simulink model "control1_flatness"  (R2023b)
settings: Solver=VariableStepAuto  StartTime=0.0  StopTime=8  RelTol=1e-3
values from neighbouring files (symbols this model uses):
  d = obs_r+threshold    (= 0.3)    [main.m]
  damping_coeff = 1/sqrt(2)    [main.m]
  initial_position = [0,r]    [main.m]
  natural_frequency = 10    [main.m]
  obs_r = 0.1    [main.m]
  obs_x = [20]    [main.m]
  obs_y = [20]    [main.m]
  parking_position = [0,0]    [main.m]
  r = 1    [main.m]
  T = 2*pi    (= 6.28318530718)    [main.m]
  t_values = 0:dt:T*1.1    [main.m]
  threshold = 0.2    [main.m]
(part 3 of 3)

== matlab function control1_flatness/Trajectory generator/Trajectory generator and obstacle detection1/Subsystem1/Whole trajectory calculation + flatness ==
  data: r input; trajectory_x output; t_values input; T input; trajectory_y output; v_d_array output; omega_d_array output; theta_d_array output; recalculate output; recalculate_obs input; d input; blending input; theta11 input; xd input; yd input; recalculate_obs1 output; old_trajectory_x input; old_trajectory_y input
function [trajectory_x, trajectory_y, v_d_array, omega_d_array, theta_d_array, recalculate,recalculate_obs1]  = fcn( r, t_values,T, recalculate_obs,d, blending, theta11, xd, yd,old_trajectory_x, old_trajectory_y)
    x0 = 0;
    y0 = 1;
    W = 2;
    H = 2;
    R = H / 2; 
    xc = x0 + W; 
    yc = y0 + R;      
    if(~recalculate_obs)
        trajectory_x = zeros(length(t_values), 1);
        trajectory_y = ones(length(t_values), 1);
        % Parameters

        
        for i = 1:length(t_values)
            t = t_values(i);
            
            if t < T/4
                % Move right
                trajectory_x(i) = x0 + (W/T*4) * t;
                trajectory_y(i) = y0;
                
            elseif t < T/2
                % Move up
                theta = -pi/2 + pi * (t - T/4) / (T/4);  % Angle from -pi/2 to pi/2
                trajectory_x(i) = xc + R * cos(theta);  % Half-circle x
                trajectory_y(i) = yc + R * sin(theta);  % Half-circle y
                
            elseif t < 3*T/4
                % Move left
                trajectory_x(i) = x0 + W - (W/T*4) * (t - T/2);
                trajectory_y(i) = y0 + H;
                
            elseif t< T
                % Move down
                trajectory_x(i) = x0;
                trajectory_y(i) = y0 + H - (H/T*4) * (t - 3*T/4);
            else
                trajectory_x(i) = x0;
                trajectory_y(i) = y0;
            end
        end

    else
        % Obstacle was detected: in the point x, y with angle theta
        center_trajectory = [x0+W/2, y0+H/2];
        % Loading previous version of the trajectory 
        % to avoid additional and useless computations of
        % previous desired path
        trajectory_x = old_trajectory_x;
        trajectory_y = old_trajectory_y;
        x1 = xd;
        y1 = yd;
        points = [trajectory_x,trajectory_y];
        [~, start_idx] = min(vecnorm(points - [x1,y1], 2, 2));

        theta1 = -theta11+pi/2;  % Adjusting the angle to get the anglefrom vertical axis (theta11 is wrt horisontal axis)

        % Estimate the obstacle location
        theta_range = linspace(theta1 - pi/4, theta1 + pi/4, 300);
        x_arc = x1 + d * sin(theta_range);
        y_arc = y1 + d * cos(theta_range);



        % Loop through the trajectory points to check for intersections

        obs_x = x1;
        obs_y = y1;
        obs_idx = start_idx;
        for i = start_idx:length(trajectory_x) - 1
            x_traj_seg = [trajectory_x(i), trajectory_x(i + 1)];
            y_traj_seg = [trajectory_y(i), trajectory_y(i + 1)];
            
            for j = 1:length(x_arc) - 1
                x_arc_seg = [x_arc(j), x_arc(j + 1)];
                y_arc_seg = [y_arc(j), y_arc(j + 1)];
                
                % Check if the two segments intersect
                [intersects, ix, iy] = segmentIntersection(x_traj_seg, y_traj_seg, x_arc_seg, y_arc_seg);
        
                if intersects
                    % Intersection found, assign coordinates
                    obs_x = ix;
                    obs_y = iy;
                    obs_idx = i;
                    break; % Exit the loop once intersection is found
                end
             end
            if obs_x ~= x1
                break; 
            end
        end
        % -- > Finding the point where the obstacle avoidance trajectory should 
        % be finished, point from which the robot should continue on
        % the regular trajectory.Creating a circle of radius d, with the 
        % center in [center_obs_x, center_obs_y].
        % After that, finding an intersection of that circle with the 
        % previous trajectory.
    
        theta_values = linspace(0, 2*pi, 500);
        x_circle = obs_x + d * cos(theta_values);
        y_circle = obs_y + d * sin(theta_values);

        % Loop through the trajectory points to check for intersections

        x2 = x1;
        y2 = y1;
        end_idx_trajectory = obs_idx;
        end_idx_circle = 1;

        for i = obs_idx:length(trajectory_x) - 1
            x_traj_seg = [trajectory_x(i), trajectory_x(i + 1)];
            y_traj_seg = [trajectory_y(i), trajectory_y(i + 1)];
            
            for j = 1:length(x_circle) - 1
                x_circle_seg = [x_circle(j), x_circle(j + 1)];
                y_circle_seg = [y_circle(j), y_circle(j + 1)];
                
                % Check if the two segments intersect
                [intersects, ix, iy] = segmentIntersection(x_traj_seg, y_traj_seg, x_circle_seg, y_circle_seg);
        
                if intersects
                    % Intersection found, assign coordinates
                    x2 = ix;
                    y2 = iy;
                    end_idx_trajectory = i;
                    end_idx_circle = j;
                    break; 
                end
            end
            if x2 ~= x1, break; end
        end

        % --> Finding the longer arc of the circle around obstacle
        % This will be the desired obstacle avoidance path
        points = [x_circle' y_circle']; % Nx2 array
        [~, idx1] = min(vecnorm(points - [x1,y1], 2, 2));
        idx2 = end_idx_circle;
        
        if idx1 < idx2
            arc1 = points(idx1:idx2, :);       
            arc2 = [points(idx2:end, :); points(1:idx1, :)];
        else
            arc1 = points(idx2:idx1, :);       
            arc2 = [points(idx1:end, :); points(1:idx2, :)];
        end
        
        idx_point1 = floor(size(arc1,1)/2);
        idx_point2 = floor(size(arc2,1)/2);
        
        distance1 = (arc1(idx_point1,1)-center_trajectory(1))^2+(arc1(idx_point1,2)-center_trajectory(2))^2;
        distance2 =  (arc2(idx_point2,1)-center_trajectory(1))^2+(arc2(idx_point2,2)-center_trajectory(2))^2;
        
        if distance1>distance2
            longer_arc = arc1;
        else
            longer_arc = arc2;
        end
        % Reverse if needed
        if(abs(longer_arc(1,1)-x1)>abs(longer_arc(1,1)-x2))
            longer_arc = flip(longer_arc);
        end


        % --> Creating a new trajectory
        idx1 = start_idx;
        idx2 = end_idx_trajectory;
        % Change of the trajectory is allowed if the ordering is okay
        % first indexwise is the point of detection and then the obstacle
        % (should always be satisfied)
        if(idx1<idx2 && t_values(idx2)<T)

            n_points = idx2 - idx1 + 1;
            total_points = size(longer_arc,1);
            indices = round(linspace(1, total_points, n_points));
            % Smoothly blend the two trajectories if needed
            trajectory_avoid_x = longer_arc(indices,1);
            trajectory_avoid_y = longer_arc(indices,2);
            trajectory_old_x = trajectory_x(idx1:idx2);
            trajectory_old_y = trajectory_y(idx1:idx2);

            trajectory_x(idx1:idx2) = blending*trajectory_avoid_x + (1-blending)*trajectory_old_x;
            trajectory_y(idx1:idx2) = blending*trajectory_avoid_y + (1-blending)*trajectory_old_y;

        end
    end

    recalculate_obs1 = 0;
    recalculate = 0;


    dt = t_values(2) - t_values(1);

    %  Derivatives
    dx_d = gradient(trajectory_x, dt);
    dy_d = gradient(trajectory_y, dt);
    ddx_d = gradient(dx_d, dt);
    ddy_d = gradient(dy_d, dt);
    
    v_d_array = sqrt(dx_d.^2 + dy_d.^2);
    omega_d_array = (ddy_d .* dx_d - ddx_d .* dy_d) ./ ((dx_d.^2 + dy_d.^2)+eps);
    theta_d_array=atan2(dy_d,dx_d);

end

== matlab function control1_flatness/One circle detection/one circle detection ==
  data: t input; x input; regulation_flag output; y input; initial_position input; regulation_flag_previous input; constant input
function regulation_flag = fcn( t, x,y,initial_position, regulation_flag_previous, constant)
if(regulation_flag_previous==0)
    if (abs(initial_position(1)- x)<0.001 && abs(initial_position(2)-y)<0.001 &&(t>constant))
        regulation_flag=1;
    else 
        regulation_flag=0;
    end
else
    regulation_flag =1;
end

== matlab function control1_flatness/Trajectory generator/Trajectory generator and obstacle detection1/Subsystem3/Triggered Subsystem/MATLAB Function1 ==
  data: t input; t_values input; trajectory_x input; x_d output; trajectory_y input; y_d output; v_d output; omega_d output; theta_d output; v_d_array input; omega_d_array input; theta_d_array input; i input; new_i output
function [x_d, y_d, v_d, omega_d, theta_d, new_i] = fcn(t, t_values, trajectory_x, trajectory_y, v_d_array, omega_d_array, theta_d_array,i)

    % When the block is not enabled (on the start),this is used to give initial position
    if (i==0)
        new_i=1;
    else
        new_i =i;
    end

    [~, idx] = min(abs(t_values - t));  % closest index to current time
    if(t>t_values(end))
        idx = length(t_values);
    end
    % Position
    x_d = trajectory_x(idx);  
    y_d = trajectory_y(idx);

    % Flatness
    v_d = v_d_array(idx);  
    omega_d = omega_d_array(idx);
    theta_d = theta_d_array(idx);

== matlab function control1_flatness/General control scheme with flatness1/Calculation of e1, e2, and e3 ==
  data: e_x input; e1 output; e_y input; e_theta input; e2 output; e3 output; theta input
function [e1,e2,e3] = fcn(e_x,e_y,e_theta,theta)
e1=e_x*cos(theta)+e_y*sin(theta);
e2=-e_x*sin(theta)+e_y*cos(theta);

if (abs(e_theta)>=2*pi)
   e_theta = mod(e_theta -2*pi, 2*pi);
end
if (abs(e_theta)>=pi)
   e_theta = mod(e_theta + pi, 2*pi)-pi;
end

e3=e_theta;
end

== matlab function control1_flatness/General control scheme with flatness1/MATLAB Function ==
  data: a input; u1 output; dam_cof input; e1 input; e2 input; e3 input; v_d input; omega_d input; u2 output
function [u1,u2] = controller(a,dam_cof,e1,e2,e3,v_d,omega_d)
k1=2*dam_cof*a
k3=k1
if abs(v_d)<1e-4
    if v_d>=0
        v_d=1e-4;
    else
        v_d=-1e-4;
    end
end
k2=(a^2-(omega_d^2))/v_d % v_d is constant for circular motion,while omega_d constant(diffrent from zero)
u1=-k1*e1;
u2=-k2*e2-k3*e3;

end

== matlab function control1_flatness/General control scheme with flatness1/MATLAB Function1 ==
  data: u1 input; v output; u2 input; v_d input; omega_d input; e3 input; omega output
function [v,omega] = input_transformation(u1,u2,v_d,omega_d,e3)
v=v_d*cos(e3)-u1;
omega=omega_d-u2;

end

== matlab function control1_flatness/General control scheme with flatness1/MATLAB Function2 ==
  data: v input; x_dot output; omega input; theta input; y_dot output; theta_dot output
function [x_dot, y_dot, theta_dot] = model(v, omega, theta)
    x_dot=v.*cos(theta);
    y_dot=v.*sin(theta);
    theta_dot = omega;
end

== matlab function control1_flatness/General control scheme with flatness1/Reset theta after -2pi to 2 ==
  data: u input; y output
function y = fcn(u)
if(u <= -2*pi+0.01)
    y = 0;
else
    y = u;
end

== matlab function control1_flatness/General control scheme with flatness1/Stopping control/Stopping condition ==
  data: v input; v_out output; omega input; t input; x input; y input; initial_position input; omega_out output; distance_treshold input
function [v_out, omega_out]= fcn(v, omega, t, x, y, initial_position, distance_treshold)

% Calculating the distance to the intial point
distance = sqrt((x - initial_position(1))^2 + (y - initial_position(2))^2);
alpha = distance/distance_treshold;

% Stopping condition to avoid the turning of the robot
% --Active when distance to the initial point is smaller than the threshold
% --Second condition is to avoid triggering this condition in the start,
%   when the robot is close to initial position
if(distance<distance_treshold && t>0.1)
    v_out = v*alpha;
    omega_out = 0;
else
    v_out = v;
    omega_out = omega;
end

== matlab function control1_flatness/Trajectory generator/Trajectory generator and obstacle detection/Subsystem1/Whole trajectory calculation + flatness ==
  data: r input; trajectory_x output; t_values input; T input; trajectory_y output; v_d_array output; omega_d_array output; theta_d_array output; recalculate output; recalculate_obs input; d input; blending input; theta11 input; xd input; yd input; recalculate_obs1 output; old_trajectory_x input; old_trajectory_y input
function [trajectory_x, trajectory_y, v_d_array, omega_d_array, theta_d_array, recalculate,recalculate_obs1]  = fcn( r, t_values,T, recalculate_obs,d, blending, theta11, xd, yd,old_trajectory_x, old_trajectory_y)
    if(~recalculate_obs)
        trajectory_x = zeros(length(t_values),1);
        trajectory_y = ones(length(t_values),1);
    
         for i = 1:length(t_values)
              t = t_values(i);
              if(t<T)
                  trajectory_x(i)= r*sin(t);
                  trajectory_y(i) = r*cos(t);
              else
                  trajectory_x(i)= r*sin(T);
                  trajectory_y(i) = r*cos(T);
              end
          end   
    else
        % Obstacle was detected: in the point x, y with angle theta

        % Loading previous version of the trajectory 
        % to avoid additional and useless computations of
        % previous desired path
        trajectory_x = old_trajectory_x;
        trajectory_y = old_trajectory_y;
        x1 = xd;
        y1 = yd;
        points = [trajectory_x,trajectory_y];
        [~, start_idx] = min(vecnorm(points - [x1,y1], 2, 2));

        theta1 = -theta11+pi/2;  % Adjusting the angle to get the anglefrom vertical axis (theta11 is wrt horisontal axis)

        % Estimate the obstacle location
        theta_range = linspace(theta1 - pi/4, theta1 + pi/4, 300);
        x_arc = x1 + d * sin(theta_range);
        y_arc = y1 + d * cos(theta_range);



        % Loop through the trajectory points to check for intersections

        obs_x = x1;
        obs_y = y1;
        obs_idx = start_idx;
        for i = start_idx:length(trajectory_x) - 1
            x_traj_seg = [trajectory_x(i), trajectory_x(i + 1)];
            y_traj_seg = [trajectory_y(i), trajectory_y(i + 1)];
            
            for j = 1:length(x_arc) - 1
                x_arc_seg = [x_arc(j), x_arc(j + 1)];
                y_arc_seg = [y_arc(j), y_arc(j + 1)];
                
                % Check if the two segments intersect
                [intersects, ix, iy] = segmentIntersection(x_traj_seg, y_traj_seg, x_arc_seg, y_arc_seg);
        
                if intersects
                    % Intersection found, assign coordinates
                    obs_x = ix;
                    obs_y = iy;
                    obs_idx = i;
                    break; % Exit the loop once intersection is found
                end
             end
            if obs_x ~= x1
                break; 
            end
        end

        % -- > Finding the point where the obstacle avoidance trajectory should 
        % be finished, point from which the robot should continue on
        % the regular trajectory.Creating a circle of radius d, with the 
        % center in [center_obs_x, center_obs_y].
        % After that, finding an intersection of that circle with the 
        % previous trajectory.

        theta_values = linspace(0, 2*pi, 500);
        x_circle = obs_x + d * cos(theta_values);
        y_circle = obs_y + d * sin(theta_values);

        % Loop through the trajectory points to check for intersections

        x2 = x1;
        y2 = y1;
        end_idx_trajectory = obs_idx;
        end_idx_circle = 1;

        for i = obs_idx:length(trajectory_x) - 1
            x_traj_seg = [trajectory_x(i), trajectory_x(i + 1)];
            y_traj_seg = [trajectory_y(i), trajectory_y(i + 1)];
            
            for j = 1:length(x_circle) - 1
                x_circle_seg = [x_circle(j), x_circle(j + 1)];
                y_circle_seg = [y_circle(j), y_circle(j + 1)];
                
                % Check if the two segments intersect
                [intersects, ix, iy] = segmentIntersection(x_traj_seg, y_traj_seg, x_circle_seg, y_circle_seg);
        
                if intersects
                    % Intersection found, assign coordinates
                    x2 = ix;
                    y2 = iy;
                    end_idx_trajectory = i;
                    end_idx_circle = j;
                    break; 
                end
            end
            if x2 ~= x1, break; end
        end

        % --> Finding the longer arc of the circle around obstacle
        % This will be the desired obstacle avoidance path
        points = [x_circle' y_circle']; % Nx2 array
        [~, idx1] = min(vecnorm(points - [x1,y1], 2, 2));
        idx2 = end_idx_circle;
        
        if idx1 < idx2
            arc1 = points(idx1:idx2, :);       
            arc2 = [points(idx2:end, :); points(1:idx1, :)];
        else
            arc1 = points(idx2:idx1, :);       
            arc2 = [points(idx1:end, :); points(1:idx2, :)];
        end
        
        idx_point1 = floor(size(arc1,1)/2);
        idx_point2 = floor(size(arc2,1)/2);
        distance1 = arc1(idx_point1,1)^2+arc1(idx_point1,2)^2;
        distance2 =  arc2(idx_point2,1)^2+arc2(idx_point2,2)^2;
        if distance1>distance2
            longer_arc = arc1;
        else
            longer_arc = arc2;
        end
        % Reverse if needed
        if(abs(longer_arc(1,1)-x1)>abs(longer_arc(1,1)-x2))
            longer_arc = flip(longer_arc);
        end


        % --> Creating a new trajectory
        idx1 = start_idx;
        idx2 = end_idx_trajectory;
        % Change of the trajectory is allowed if the ordering is okay
        % first indexwise is the point of detection and then the obstacle
        % (should always be satisfied)
        if(idx1<idx2 && t_values(idx2)<T)

            n_points = idx2 - idx1 + 1;
            total_points = size(longer_arc,1);
            indices = round(linspace(1, total_points, n_points));
            % Smoothly blend the two trajectories if needed
            trajectory_avoid_x = longer_arc(indices,1);
            trajectory_avoid_y = longer_arc(indices,2);
            trajectory_old_x = trajectory_x(idx1:idx2);
            trajectory_old_y = trajectory_y(idx1:idx2);

            trajectory_x(idx1:idx2) = blending*trajectory_avoid_x + (1-blending)*trajectory_old_x;
            trajectory_y(idx1:idx2) = blending*trajectory_avoid_y + (1-blending)*trajectory_old_y;

        end
    end

    recalculate_obs1 = 0;
    recalculate = 0;


    dt = t_values(2) - t_values(1);

    %  Derivatives
    dx_d = gradient(trajectory_x, dt);
    dy_d = gradient(trajectory_y, dt);
    ddx_d = gradient(dx_d, dt);
    ddy_d = gradient(dy_d, dt);
    
    v_d_array = sqrt(dx_d.^2 + dy_d.^2);
    omega_d_array = (ddy_d .* dx_d - ddx_d .* dy_d) ./ ((dx_d.^2 + dy_d.^2)+eps);
    theta_d_array=atan2(dy_d,dx_d);

end

== matlab function control1_flatness/Trajectory generator/Trajectory generator and obstacle detection/MATLAB Function ==
  data: initial_position input; x1 input; y1 input; v1 input; omega1 input; theta1 input; i input; x output; y output; v output; omega output; theta output
function [x,y,v,omega,theta] = fcn(initial_position, x1,y1,v1, omega1, theta1,i)

if(i == 0)
    x = initial_position(1);
    y = initial_position(2);
    v = 0;
    omega = 0;
    theta=0;
else
    x = x1;
    y = y1;
    v = v1;
    omega = omega1;
    theta=theta1;
end

== matlab function control1_flatness/Trajectory generator/Trajectory generator and obstacle detection2/MATLAB Function ==
  data: initial_position input; x1 input; y1 input; v1 input; omega1 input; theta1 input; i input; x output; y output; v output; omega output; theta output
function [x,y,v,omega,theta] = fcn(initial_position, x1,y1,v1, omega1, theta1,i)

if(i == 0)
    x = initial_position(1);
    y = initial_position(2);
    v = 0;
    omega = 0;
    theta=0;
else
    x = x1;
    y = y1;
    v = v1;
    omega = omega1;
    theta=theta1;
end
